simulink model "first"  (R2023b)
settings: Solver=FixedStepAuto  StartTime=0.0  StopTime=10  FixedStep=0.01  RelTol=1e-3
undefined symbols (not defined in the file): A, B, K, Kl, Km, Q, R, x0
settings Model: Creator=evdokiiagalkina  LastModifiedBy=evdokiiagalkina

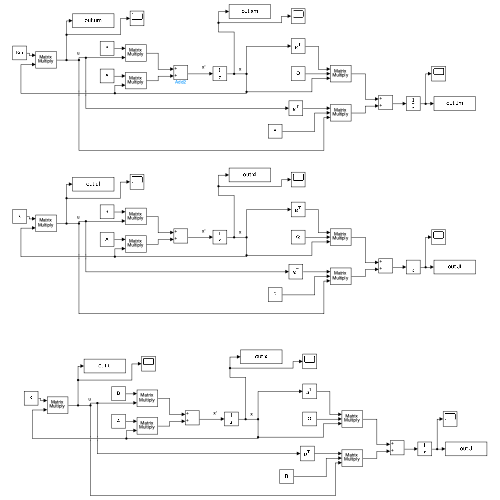
[thumbnail: Simulink's stored preview of the top-level diagram]
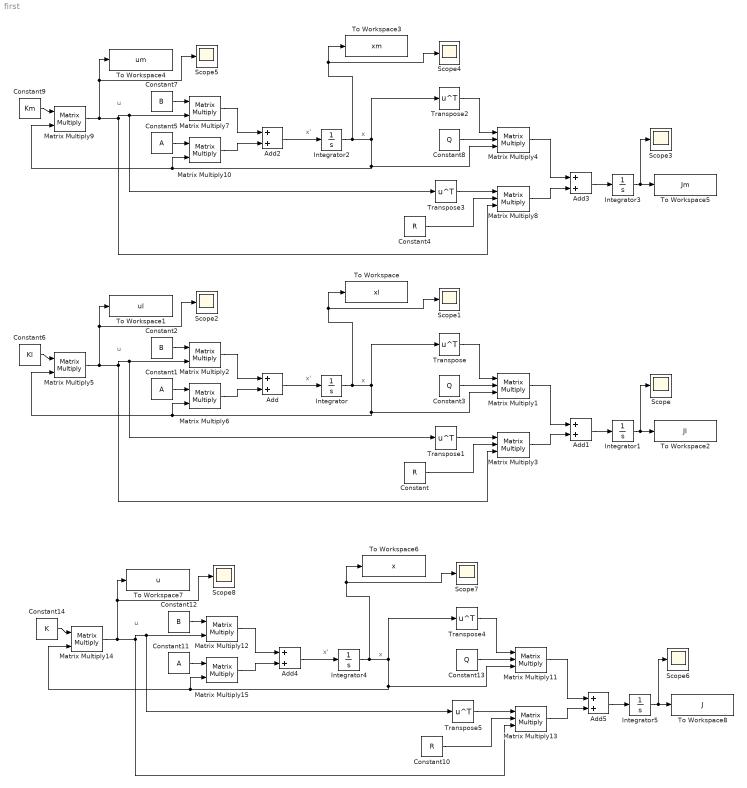
== system first ==
  note: u
  note: x
  note: x'
  note: x'
  note: u
  note: x
  note: x'
  note: u
  note: x
  Add{,1..5} (6 alike) : Sum
  Constant : Constant  Value=R  VectorParams1D=off
  Constant1 : Constant  Value=A
  Constant10 : Constant  Value=R  VectorParams1D=off
  Constant11 : Constant  Value=A
  Constant12 : Constant  Value=B
  Constant13 : Constant  Value=Q  VectorParams1D=off
  Constant14 : Constant  Value=K  VectorParams1D=off
  Constant2 : Constant  Value=B
  Constant3 : Constant  Value=Q  VectorParams1D=off
  Constant4 : Constant  Value=R  VectorParams1D=off
  Constant5 : Constant  Value=A
  Constant6 : Constant  Value=Kl  VectorParams1D=off
  Constant7 : Constant  Value=B
  Constant8 : Constant  Value=Q  VectorParams1D=off
  Constant9 : Constant  Value=Km  VectorParams1D=off
  Integrator : Integrator  InitialCondition=x0  IgnoreLimit=on
  Integrator1 : Integrator
  Integrator2 : Integrator  InitialCondition=x0  IgnoreLimit=on
  Integrator3 : Integrator
  Integrator4 : Integrator  InitialCondition=x0  IgnoreLimit=on
  Integrator5 : Integrator
  Matrix Multiply{1,3..4,8,11,13} (6 alike) : Product  Inputs=3  Multiplication=Matrix(*)
  Matrix Multiply{2,5..7,9..10,12,14..15} (9 alike) : Product  Multiplication=Matrix(*)
  Scope{,1..8} (9 alike) : Scope
  To Workspace : ToWorkspace  VariableName=xl  SaveFormat=Timeseries  SampleTime=-1
  To Workspace1 : ToWorkspace  VariableName=ul  SaveFormat=Timeseries  SampleTime=-1
  To Workspace2 : ToWorkspace  VariableName=Jl  SaveFormat=Timeseries  SampleTime=-1
  To Workspace3 : ToWorkspace  VariableName=xm  SaveFormat=Timeseries  SampleTime=-1
      settings: Save2DSignal=2-D array (concatenate along first dimension)
  To Workspace4 : ToWorkspace  VariableName=um  SaveFormat=Timeseries  SampleTime=-1
  To Workspace5 : ToWorkspace  VariableName=Jm  SaveFormat=Timeseries  SampleTime=-1
  To Workspace6 : ToWorkspace  VariableName=x  SaveFormat=Timeseries  SampleTime=-1
  To Workspace7 : ToWorkspace  VariableName=u  SaveFormat=Timeseries  SampleTime=-1
  To Workspace8 : ToWorkspace  VariableName=J  SaveFormat=Timeseries  SampleTime=-1
  Transpose{,1..5} (6 alike) : Math  Operator=transpose
  wires:
  Constant2/1 -> Matrix Multiply2/1
  Matrix Multiply6/1 -> Add/2
  Matrix Multiply5/1 -> Scope2/1, To Workspace1/1, Transpose1/1, Matrix Multiply2/2, Matrix Multiply3/3
  Integrator/1 -> Scope1/1, To Workspace/1, Matrix Multiply1/3, Matrix Multiply6/2, Matrix Multiply5/2, Transpose/1
  Add/1 -> Integrator/1
  Matrix Multiply2/1 -> Add/1
  Constant1/1 -> Matrix Multiply6/1
  Constant6/1 -> Matrix Multiply5/1
  Integrator1/1 -> Scope/1, To Workspace2/1
  Add1/1 -> Integrator1/1
  Matrix Multiply1/1 -> Add1/1
  Matrix Multiply3/1 -> Add1/2
  Constant/1 -> Matrix Multiply3/2
  Constant3/1 -> Matrix Multiply1/2
  Transpose/1 -> Matrix Multiply1/1
  Transpose1/1 -> Matrix Multiply3/1
  Transpose2/1 -> Matrix Multiply4/1
  Constant8/1 -> Matrix Multiply4/2
  Constant4/1 -> Matrix Multiply8/2
  Add3/1 -> Integrator3/1
  Transpose3/1 -> Matrix Multiply8/1
  Matrix Multiply8/1 -> Add3/2
  Matrix Multiply7/1 -> Add2/1
  Integrator3/1 -> Scope3/1, To Workspace5/1
  Matrix Multiply4/1 -> Add3/1
  Constant7/1 -> Matrix Multiply7/1
  Matrix Multiply10/1 -> Add2/2
  Matrix Multiply9/1 -> Scope5/1, To Workspace4/1, Transpose3/1, Matrix Multiply7/2, Matrix Multiply8/3
  Integrator2/1 -> Scope4/1, To Workspace3/1, Matrix Multiply4/3, Matrix Multiply10/2, Matrix Multiply9/2, Transpose2/1
  Add2/1 -> Integrator2/1
  Constant5/1 -> Matrix Multiply10/1
  Constant9/1 -> Matrix Multiply9/1
  Transpose4/1 -> Matrix Multiply11/1
  Constant13/1 -> Matrix Multiply11/2
  Constant10/1 -> Matrix Multiply13/2
  Add5/1 -> Integrator5/1
  Transpose5/1 -> Matrix Multiply13/1
  Matrix Multiply13/1 -> Add5/2
  Matrix Multiply12/1 -> Add4/1
  Integrator5/1 -> Scope6/1, To Workspace8/1
  Matrix Multiply11/1 -> Add5/1
  Constant12/1 -> Matrix Multiply12/1
  Matrix Multiply15/1 -> Add4/2
  Matrix Multiply14/1 -> Scope8/1, To Workspace7/1, Transpose5/1, Matrix Multiply12/2, Matrix Multiply13/3
  Integrator4/1 -> Scope7/1, To Workspace6/1, Matrix Multiply11/3, Matrix Multiply15/2, Matrix Multiply14/2, Transpose4/1
  Add4/1 -> Integrator4/1
  Constant11/1 -> Matrix Multiply15/1
  Constant14/1 -> Matrix Multiply14/1
